simulink model "IntegrationTestSim"  (R2018b)
settings: Solver=ode45  StartTime=0.0  StopTime=600  RelTol=1e-3  EnableMultiTasking=on
values from neighbouring files (symbols this model uses):
  enableHorzMan = 1    [IntegrationTestClass.m]
  enableVertMan = 0    [IntegrationTestClass.m]
  ignorePrevAlert = 1    [IntegrationTestClass.m]
  sim_sampleTime = 0.1    [IntegrationTestClass.m]
  uasSensorSelected = 1    [IntegrationTestClass.m]
  uasSurveillance_sampleTime = 0.1    [IntegrationTestClass.m]
undefined symbols (not defined in the file or in its folder): ac1dyn_alt0_ft, ac1dyn_lat0_rad, ac1dyn_lon0_rad, daa_turnRate_dps, daa_vertRate_fpm, dh_flag, dh_ftps, dpsi_flag, dpsi_radps, uasPilot_altitudeK, uasPilot_altitudeOffset, uasPilot_altitudeTheta, uasPilot_coordDelayK, uasPilot_coordDelayMin, uasPilot_coordDelayTheta, uasPilot_desiredTurnRate_dps, uasPilot_desiredVertRate_ftpm, uasPilot_deterministicMode, uasPilot_dt_s, uasPilot_executionDelayMin, uasPilot_executionDelayMu, uasPilot_initialDelayMin, uasPilot_initialDelayMu, uasPilot_maxRelativeHdg, uasPilot_meanUpdateTimes, uasPilot_mentalFilter_climbThresh_fps, uasPilot_mentalFilter_numSamp, uasPilot_mentalFilter_turnThresh_rad, uasPilot_minUpdateTimes, uasPilot_operatorEnabled, uasPilot_probDescend, uasPilot_probFollowMinDev, uasPilot_probLeftTurn, uasPilot_probTurn, uasPilot_reducedClimbAlt_ft, uasPilot_reducedTurnAngle_deg, uasPilot_seedChoose, uasPilot_seedCoordDelay, uasPilot_seedExecutionDelay, uasPilot_seedInitialDelay, uasPilot_seedTurn, uasPilot_seedUpdate, uasPilot_seedVertical, uasPilot_triggerLevel, uasPilot_turnK, uasPilot_turnOffset, uasPilot_turnTheta
libraries: simulink x4, BasicAircraftDynamicsBlock x3, NominalTrajectory x2, FlattenAircraftEstimateBus x2, PerfectSurveillanceBlock x2, sph2cart x2, DaidalusV201Block x1, HysteresisFilterBlock x1, MofNFilterBlock x1, CommonMetricsBlock x1, SLoWCBlock x1, WellClearMetricsBlock x1
(part 1 of 3)
settings Model: Creator=JO20596  LastModifiedBy=BI28030
settings DataIOCC: LimitDataPoints=on  MaxDataPoints=10000  SignalLoggingSaveFormat=ModelDataLogs  SaveState=on  StateSaveName=xoutNew  OutputSaveName=youtNew
settings OptimizationCC: ExpressionDepthLimit=2147483647  LifeSpan=inf
settings DebuggingCC: UnderspecifiedInitializationDetection=Classic  MergeDetectMultiDrivingBlocksExec=none  SolverPrmCheckMsg=warning  FcnCallInpInsideContextMsg=warning  StateNameClashWarn=warning  SFUnexpectedBacktrackingDiag=warning  SFNoUnconditionalDefaultTransitionDiag=warning  SFExecutionAtInitializationDiag=none
settings HardwareCC: ProdBitPerPointer=32  ProdBitPerSizeT=32  ProdBitPerPtrDiffT=32  ProdLargestAtomicFloat=None  ProdIntDivRoundTo=Undefined  ProdEndianess=Unspecified  ProdWordSize=32  ProdHWDeviceType=32-bit Generic
settings ModelReferenceCC: PropagateSignalLabelsOutOfModel=off
settings SFSimCC: SimUseLocalCustomCode=off
settings RTWCC: RTWUseLocalCustomCode=off
settings CodeAppCC: StateflowObjectComments=on
settings GRTTargetCC: TargetLangStandard=C89/C90 (ANSI)  GeneratePreprocessorConditionals=Disable all  CombineOutputUpdateFcns=off  GRTInterface=on
settings ConfigComp: CovMetricSettings=dw  CovHtmlReporting=on  CovSaveCumulativeToWorkspaceVar=on  CovSaveSingleToWorkspaceVar=on  CovExternalEMLEnable=off

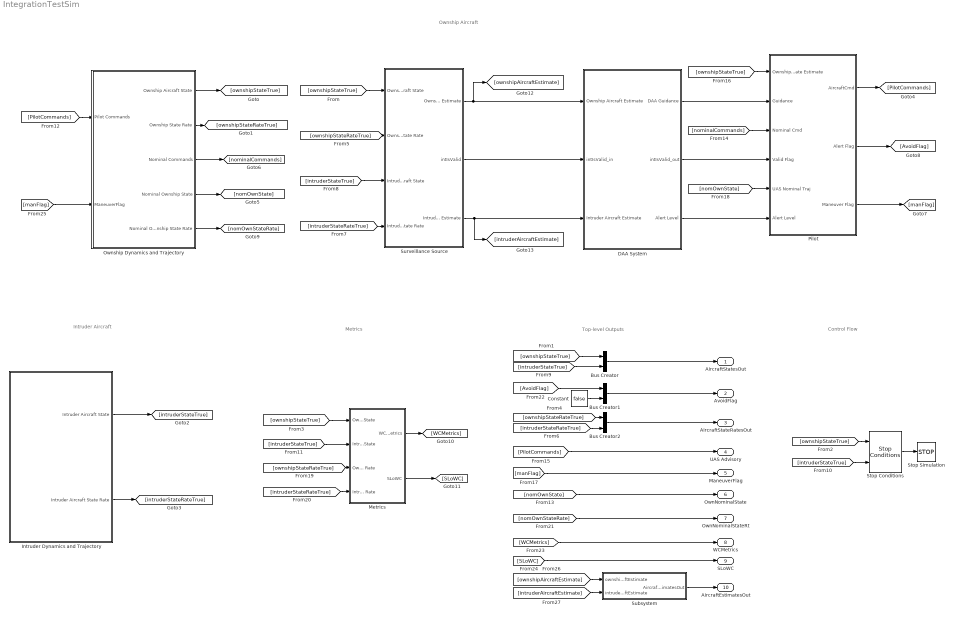
== system IntegrationTestSim ==
  note: Metrics
  note: Control Flow
  note: Top-level Outputs
  note: Ownship Aircraft
  note: Intruder Aircraft
  Bus Creator : BusCreator  Inputs=2
  Bus Creator1 : BusCreator  Inputs=2
  Bus Creator2 : BusCreator  Inputs=2
  Constant : Constant  Value=false  SampleTime=sim_sampleTime
  DAA System : Subsystem
  Intruder Dynamics and Trajectory : Subsystem
  Metrics : Subsystem
  Ownship Dynamics and Trajectory : Subsystem
  Pilot : Subsystem  mask(Heuristic Operator Model){dt=uasPilot_dt_s, operator_enabled=uasPilot_operatorEnabled, deterministicMode=uasPilot_deterministicMode, trigger_level=uasPilot_triggerLevel, mean_initial_delay=uasPilot_initialDelayMu, min_initial_delay=uasPilot_initialDelayMin, coord_delay_k=uasPilot_coordDelayK, coord_delay_theta=uasPilot_coordDelayTheta, coord_delay_min=uasPilot_coordDelayMin, mean_exec_delay=uasPilot_executionDelayMu, min_exec_delay=uasPilot_executionDelayMin, min_upd_times=uasPilot_minUpdateTimes, mean_upd_times=uasPilot_meanUpdateTimes, rng_seed_initial=uasPilot_seedInitialDelay, rng_seed_coord=uasPilot_seedCoordDelay, rng_seed_execution=uasPilot_seedExecutionDelay, rng_seed_update=uasPilot_seedUpdate, prob_follow_min=uasPilot_probFollowMinDev, prob_turn_left=uasPilot_probLeftTurn, prob_descend=uasPilot_probDescend, prob_turn=uasPilot_probTurn, max_hdg_diff=uasPilot_maxRelativeHdg, turn_k=uasPilot_turnK, turn_theta=uasPilot_turnTheta, turn_offset=uasPilot_turnOffset, alt_k=uasPilot_altitudeK, alt_theta=uasPilot_altitudeTheta, alt_offset=uasPilot_altitudeOffset, rng_seed_horz=uasPilot_seedTurn, rng_seed_vert=uasPilot_seedVertical, rng_seed_horz_vs_vert=uasPilot_seedChoose, max_turn_rate=uasPilot_desiredTurnRate_dps, settle_angle=uasPilot_reducedTurnAngle_deg, max_vert_rate=uasPilot_desiredVertRate_ftpm, settle_dist=uasPilot_reducedClimbAlt_ft, mental_filter_samples=uasPilot_mentalFilter_numSamp, mental_filter_turn_thresh=uasPilot_mentalFilter_turnThresh_rad, mental_filter_climb_thresh=uasPilot_mentalFilter_climbThresh_fps, daa_turnRate=daa_turnRate_dps, daa_vertRate=daa_vertRate_fpm}
      mask prompts: dt "Sample Time"; operator_enabled "Enable Pilot Response?"; deterministicMode "Deterministic Mode?"; trigger_level "Trigger Alert Level"; mean_initial_delay "Mean Initial Delay"; min_initial_delay "Minimum Initial Delay"; coord_delay_k "Coordination Delay Shape Parameter (k)"; coord_delay_theta "Coordination Delay Scale Parameter (theta)"; coord_delay_min "Minimum Coordination Delay"; mean_exec_delay "Mean Execution Delay"; min_exec_delay "Minimum Execution Delay"; min_upd_times "Minimum Maneuver Update Times by Alert Level"; mean_upd_times "Mean Maneuver Update Times by Alert Level (sec)"; rng_seed_initial "Random Seed (Initial Delay)"; rng_seed_coord "Random Seed (Coordiantion Delay)"; rng_seed_execution "Random Seed (Execution Delay)"; rng_seed_update "Random Seed (Update Decision)"; prob_follow_min "Probability of Following Minimum Turn"; prob_turn_left "Probability of Turning Left vs. Right"; prob_descend "Probability of Descend vs. CLimb"; prob_turn "Probability of Choosing Turn"; max_hdg_diff "Maximum Heading Difference to Override"; turn_k "Turn Magnitude Shape Parameter (k)"; turn_theta "Turn Magnitude Scale Parameter (theta)"; turn_offset "Turn Magnitude Offset"; alt_k "Altitude Shape Parameter (k)"; alt_theta "Altitude Scale Parameter (theta)"; alt_offset "Altitude Offset"; rng_seed_horz "Random Seed (Horizontal Maneuver Choice)"; rng_seed_vert "Random Seed (Vertical Maneuver Choice)"; rng_seed_horz_vs_vert "Random Seed (Turn vs. Climb)"; max_turn_rate "Desired Turn Rate (deg/s)"; settle_angle "Angle from Desired Heading to Begin Settle (deg)"; max_vert_rate "Desired Vertical Rate (ft/min)"; settle_dist "Distance from Desired Altitude to Begin Settle (ft)"; mental_filter_samples "Number of Samples for Mental Filter"; mental_filter_turn_thresh "Mental Filter Turn Threshold (rad)"; mental_filter_climb_thresh "Mental Filter Climb Threshold (fps)"; daa_turnRate "Max Turn Rate (deg/s)"; daa_vertRate "Max Vertical Rate (fpm)"
      mask help: Identifies pilot response to surveillance estimates of intruder position/course. Either a horizontal or vertical maneuver to maintain well clear.
      mask DialogControl ParameterTabVar0 Prompt: Tab
      mask DialogControl ParameterTabVar01 Prompt: Alert
      mask DialogControl ParameterTabVar012 Prompt: Maneuver Timing
      mask DialogControl ParameterTabVar0123 Prompt: Maneuver Selection
      mask DialogControl ParameterTabVar01234 Prompt: Maneuver Dynamics
      mask DialogControl Container12 Prompt: Pilot Mental Filter
      mask DialogControl Container11 Prompt: DAIDALUS Parameters
  Stop Conditions : StopConditionsBlock/Stop Conditions  range_limit_ft=stop_range_ft  altitude_limit_ft=stop_altitude_ft
  Stop Simulation : Stop
  Subsystem : Subsystem
  Surveillance Source : Subsystem
  AircraftStatesOut : Outport
  AvoidFlag : Outport  Port=2
  AircraftStateRatesOut : Outport  Port=3
  UAS Advisory : Outport  Port=4
  ManeuverFlag : Outport  Port=5
  OwnNominalState : Outport  Port=6
  OwnNominalStateRt : Outport  Port=7
  WCMetrics : Outport  Port=8
  SLoWC : Outport  Port=9
  AircraftEstimatesOut : Outport  Port=10
  wires:
  Bus Creator1/1 -> AvoidFlag/1
  Bus Creator2/1 -> AircraftStateRatesOut/1
  Constant/1 -> Bus Creator1/2
  [AvoidFlag] -> Bus Creator1/1
  Stop Conditions/1 -> Stop Simulation/1
  Bus Creator/1 -> AircraftStatesOut/1
  [ownshipStateTrue] -> Surveillance Source/1(Ownship Aircraft State)
  [ownshipStateTrue] -> Bus Creator/1
  [ownshipStateTrue] -> Stop Conditions/1
  [ownshipStateRateTrue] -> Bus Creator2/1
  [ownshipStateRateTrue] -> Surveillance Source/2(Ownship Aircraft State Rate)
  [intruderStateRateTrue] -> Bus Creator2/2
  [intruderStateRateTrue] -> Surveillance Source/4(Intruder Aircraft State Rate)
  [intruderStateTrue] -> Surveillance Source/3(Intruder Aircraft State)
  [intruderStateTrue] -> Bus Creator/2
  [intruderStateTrue] -> Stop Conditions/2
  Pilot/1(AircraftCmd) -> [PilotCommands]
  DAA System/1(DAA Guidance) -> Pilot/2(Guidance)
  DAA System/3(Alert Level) -> Pilot/6(Alert Level)
  [nomOwnState] -> Pilot/5(UAS Nominal Traj)
  [nominalCommands] -> Pilot/3(Nominal Cmd)
  DAA System/2(intIsValid_out) -> Pilot/4(Valid Flag)
  Surveillance Source/1(Ownship Aircraft Estimate) -> [ownshipAircraftEstimate], DAA System/1(Ownship Aircraft Estimate)
  Surveillance Source/2(intIsValid) -> DAA System/2(intIsValid_in)
  Surveillance Source/3(Intruder Aircraft Estimate) -> [intruderAircraftEstimate], DAA System/3(Intruder Aircraft Estimate)
  [ownshipStateTrue] -> Pilot/1(Ownship State Estimate)
  [PilotCommands] -> UAS Advisory/1
  Pilot/3(Maneuver Flag) -> [manFlag]
  [manFlag] -> ManeuverFlag/1
  [ownshipStateTrue] -> Metrics/1(Ownship State)
  [intruderStateTrue] -> Metrics/2(Intruder State)
  Pilot/2(Alert Flag) -> [AvoidFlag]
  [ownshipStateRateTrue] -> Metrics/3(Ownship State Rate)
  [intruderStateRateTrue] -> Metrics/4(Intruder State Rate)
  [nomOwnState] -> OwnNominalState/1
  [nomOwnStateRate] -> OwnNominalStateRt/1
  Metrics/1(WCMetrics) -> [WCMetrics]
  Metrics/2(SLoWC) -> [SLoWC]
  [WCMetrics] -> WCMetrics/1
  [SLoWC] -> SLoWC/1
  [PilotCommands] -> Ownship Dynamics and Trajectory/1(Pilot Commands)
  Ownship Dynamics and Trajectory/1(Ownship Aircraft State) -> [ownshipStateTrue]
  Ownship Dynamics and Trajectory/2(Ownship State Rate) -> [ownshipStateRateTrue]
  Ownship Dynamics and Trajectory/3(Nominal Commands) -> [nominalCommands]
  Ownship Dynamics and Trajectory/4(Nominal Ownship State) -> [nomOwnState]
  Ownship Dynamics and Trajectory/5(Nominal Ownship State Rate) -> [nomOwnStateRate]
  Intruder Dynamics and Trajectory/1(Intruder Aircraft State) -> [intruderStateTrue]
  Intruder Dynamics and Trajectory/2(Intruder Aircraft State Rate) -> [intruderStateRateTrue]
  [manFlag] -> Ownship Dynamics and Trajectory/2(ManeuverFlag)
  [ownshipAircraftEstimate] -> Subsystem/1(ownshipAircraftEstimate)
  [intruderAircraftEstimate] -> Subsystem/2(intruderAircraftEstimate)
  Subsystem/1(AircraftEstimatesOut) -> AircraftEstimatesOut/1

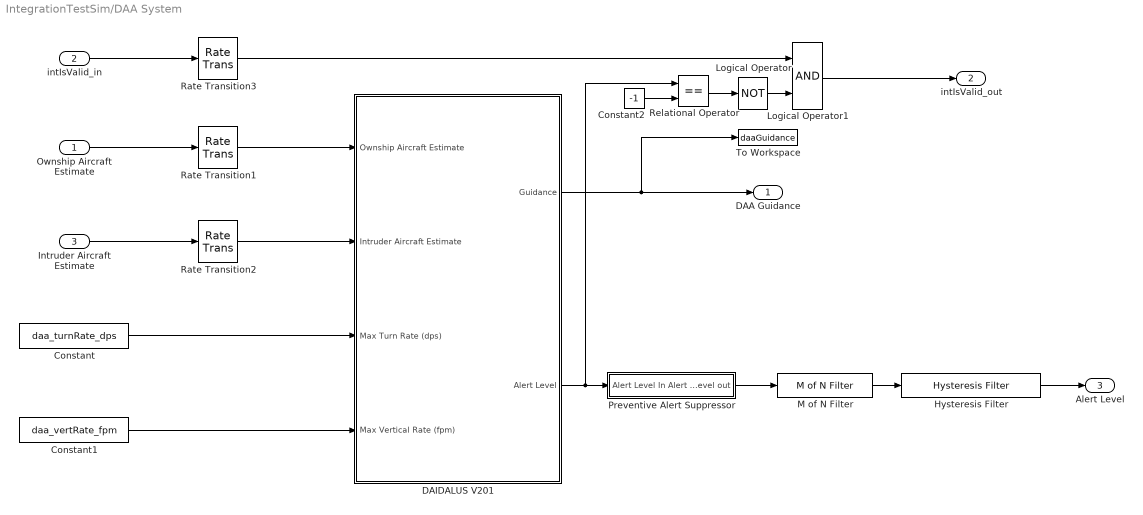
== system IntegrationTestSim/DAA System ==
  Ownship Aircraft Estimate : Inport
  intIsValid_in : Inport  Port=2
  Intruder Aircraft Estimate : Inport  Port=3
  Constant : Constant  Value=daa_turnRate_dps
  Constant1 : Constant  Value=daa_vertRate_fpm
  Constant2 : Constant  Value=-1
  DAIDALUS V201 : Subsystem
  Hysteresis Filter : HysteresisFilterBlock/Hysteresis Filter  signal_hold_time=ac1AlertHyst_signalHoldTime
  Logical Operator : Logic  Operator=NOT  AllPortsSameDT=off  OutDataTypeStr=boolean
  Logical Operator1 : Logic  AllPortsSameDT=off  OutDataTypeStr=boolean
  M of N Filter : MofNFilterBlock/M of N Filter  num_samples=ac1AlertMofN_numSamples  num_upgrade=ac1AlertMofN_numSamplesUp  num_downgrade=ac1AlertMofN_numSamplesDown
  Preventive Alert Suppressor : Subsystem
  Rate Transition1 : RateTransition  OutPortSampleTime=uasLogic_sampleTime
  Rate Transition2 : RateTransition  OutPortSampleTime=uasLogic_sampleTime
  Rate Transition3 : RateTransition  OutPortSampleTime=uasLogic_sampleTime
  Relational Operator : RelationalOperator  Operator===  OutDataTypeStr=boolean  RndMeth=Simplest
  To Workspace : ToWorkspace  VariableName=daaGuidance  SampleTime=-1
  DAA Guidance : Outport
  intIsValid_out : Outport  Port=2
  Alert Level : Outport  Port=3
  wires:
  Ownship Aircraft Estimate/1 -> Rate Transition1/1
  Intruder Aircraft Estimate/1 -> Rate Transition2/1
  DAIDALUS V201/2(Alert Level) -> Relational Operator/1, Preventive Alert Suppressor/1(Alert Level In)
  Constant/1 -> DAIDALUS V201/3(Max Turn Rate (dps))
  Constant1/1 -> DAIDALUS V201/4(Max Vertical Rate (fpm))
  DAIDALUS V201/1(Guidance) -> To Workspace/1, DAA Guidance/1
  Hysteresis Filter/1 -> Alert Level/1
  Preventive Alert Suppressor/1(Alert Level out) -> M of N Filter/1
  intIsValid_in/1 -> Rate Transition3/1
  Rate Transition1/1 -> DAIDALUS V201/1(Ownship Aircraft Estimate)
  Rate Transition2/1 -> DAIDALUS V201/2(Intruder Aircraft Estimate)
  M of N Filter/1 -> Hysteresis Filter/1
  Constant2/1 -> Relational Operator/2
  Relational Operator/1 -> Logical Operator/1
  Logical Operator/1 -> Logical Operator1/2
  Logical Operator1/1 -> intIsValid_out/1
  Rate Transition3/1 -> Logical Operator1/1

== system IntegrationTestSim/Intruder Dynamics and Trajectory ==
  AC2 - Nominal Trajectory : NominalTrajectory/Nominal Trajectory  eventFilename=event2.mat  ts=.1
  Basic Aircraft Dynamics : BasicAircraftDynamicsBlock/Basic Aircraft Dynamics  ts_dynamics=.1  v_ftps_0=ac2dyn_v_ftps  N_ft_0=ac2dyn_N_ft  E_ft_0=ac2dyn_E_ft  h_ft_0=ac2dyn_h_ft  psi_rad_0=ac2dyn_psi_rad  theta_rad_0=ac2dyn_theta_rad  phi_rad_0=ac2dyn_phi_rad  a_ftpss_0=ac2dyn_a_ftpss  v_ftps_max=ac2dyn_con.maxAirspeed_ftps  v_ftps_min=ac2dyn_con.minAirspeed_ftps  dv_ftpss_max=ac2dyn_con.maxAcceleration_ftpss  dv_ftpss_min=ac2dyn_con.minAcceleration_ftpss  dh_ftps_max=ac2dyn_con.maxVerticalRate_ftps  dh_ftps_min=ac2dyn_con.minVerticalRate_ftps  q_radps_max=ac2dyn_con.maxPitchRate_radps  phi_rad_max=ac2dyn_con.maxBankAngle_rad  dphi_radps_max=ac2dyn_con.maxRollRate_radps  r_radps_max=ac2dyn_con.maxYawRate_radps  pNUM=ac2dyn_con.dynamicsNumeratorRollRate  pDEN=ac2dyn_con.dynamicsDenominatorRollRate  hNUM=ac2dyn_con.dynamicsNumeratorVerticalRate  hDEN=ac2dyn_con.dynamicsDenominatorVerticalRate  rNUM=ac2dyn_con.dynamicsNumeratorYawRate  rDEN=ac2dyn_con.dynamicsDenominatorYawRate  lat0_rad=ac2dyn_lat0_rad  lon0_rad=ac2dyn_lon0_rad  alt_ft=ac2dyn_alt0_ft
  Terminator1 : Terminator
  Intruder Aircraft State : Outport
  Intruder Aircraft State Rate : Outport  Port=2
  wires:
  Basic Aircraft Dynamics/2 -> Terminator1/1
  Basic Aircraft Dynamics/1 -> Intruder Aircraft State/1  "Aircraft2"
  AC2 - Nominal Trajectory/1 -> Basic Aircraft Dynamics/1
  Basic Aircraft Dynamics/3 -> Intruder Aircraft State Rate/1

== system IntegrationTestSim/Metrics ==
  Ownship State : Inport
  Intruder State : Inport  Port=2
  Ownship State Rate : Inport  Port=3
  Intruder State Rate : Inport  Port=4
  Common Metrics : CommonMetricsBlock/Common Metrics
  Compute SLoWC : Subsystem  mask{DMOD=4000, tauMod=35, altDiff=450}
      mask prompts: altDiff "Altitude Difference Threshold:"
  Well Clear Metrics : Subsystem
  WCMetrics : Outport
  SLoWC : Outport  Port=2
  wires:
  Ownship State/1 -> Common Metrics/1, Well Clear Metrics/1(ownState), Compute SLoWC/1(ownState)
  Intruder State/1 -> Common Metrics/2, Well Clear Metrics/2(intState), Compute SLoWC/2(intState)
  Ownship State Rate/1 -> Well Clear Metrics/3(ownStateRate), Compute SLoWC/3(ownStateRate)
  Intruder State Rate/1 -> Well Clear Metrics/4(intStateRate), Compute SLoWC/4(intStateRate)
  Well Clear Metrics/1(WCV_MIT) -> WCMetrics/1
  Compute SLoWC/1(SLoWC) -> SLoWC/1

== system IntegrationTestSim/Ownship Dynamics and Trajectory ==
  Pilot Commands : Inport
  ManeuverFlag : Inport  Port=2
  Basic Aircraft Dynamics : BasicAircraftDynamicsBlock/Basic Aircraft Dynamics  ts_dynamics=.1  v_ftps_0=ac1dyn_v_ftps  N_ft_0=ac1dyn_N_ft  E_ft_0=ac1dyn_E_ft  h_ft_0=ac1dyn_h_ft  psi_rad_0=ac1dyn_psi_rad  theta_rad_0=ac1dyn_theta_rad  phi_rad_0=ac1dyn_phi_rad  a_ftpss_0=ac1dyn_a_ftpss  v_ftps_max=ac1dyn_con.maxAirspeed_ftps  v_ftps_min=ac1dyn_con.minAirspeed_ftps  dv_ftpss_max=ac1dyn_con.maxAcceleration_ftpss  dv_ftpss_min=ac1dyn_con.minAcceleration_ftpss  dh_ftps_max=ac1dyn_con.maxVerticalRate_ftps  dh_ftps_min=ac1dyn_con.minVerticalRate_ftps  q_radps_max=ac1dyn_con.maxPitchRate_radps  phi_rad_max=ac1dyn_con.maxBankAngle_rad  dphi_radps_max=ac1dyn_con.maxRollRate_radps  r_radps_max=ac1dyn_con.maxYawRate_radps  pNUM=ac1dyn_con.dynamicsNumeratorRollRate  pDEN=ac1dyn_con.dynamicsDenominatorRollRate  hNUM=ac1dyn_con.dynamicsNumeratorVerticalRate  hDEN=ac1dyn_con.dynamicsDenominatorVerticalRate  rNUM=ac1dyn_con.dynamicsNumeratorYawRate  rDEN=ac1dyn_con.dynamicsDenominatorYawRate  lat0_rad=ac2dyn_lat0_rad  lon0_rad=ac2dyn_lon0_rad  alt_ft=ac2dyn_alt0_ft
  Multiport Switch : MultiPortSwitch  DataPortOrder=Specify indices  DataPortIndices={1,0}
  Nominal Commands and Trajectory : Subsystem
  Terminator : Terminator
  Ownship Aircraft State : Outport
  Ownship State Rate : Outport  Port=2
  Nominal Commands : Outport  Port=3
  Nominal Ownship State : Outport  Port=4
  Nominal Ownship State Rate : Outport  Port=5
  wires:
  Nominal Commands and Trajectory/3(NominalOwnshipStateRate) -> Nominal Ownship State Rate/1
  Basic Aircraft Dynamics/1 -> Ownship Aircraft State/1  "Aircraft1"
  Nominal Commands and Trajectory/1(Nominal Commands) -> Nominal Commands/1, Multiport Switch/3
  Basic Aircraft Dynamics/3 -> Ownship State Rate/1
  Nominal Commands and Trajectory/2(NominalOwnshipState) -> Nominal Ownship State/1
  Basic Aircraft Dynamics/2 -> Terminator/1
  ManeuverFlag/1 -> Multiport Switch/1
  Multiport Switch/1 -> Basic Aircraft Dynamics/1
  Pilot Commands/1 -> Multiport Switch/2

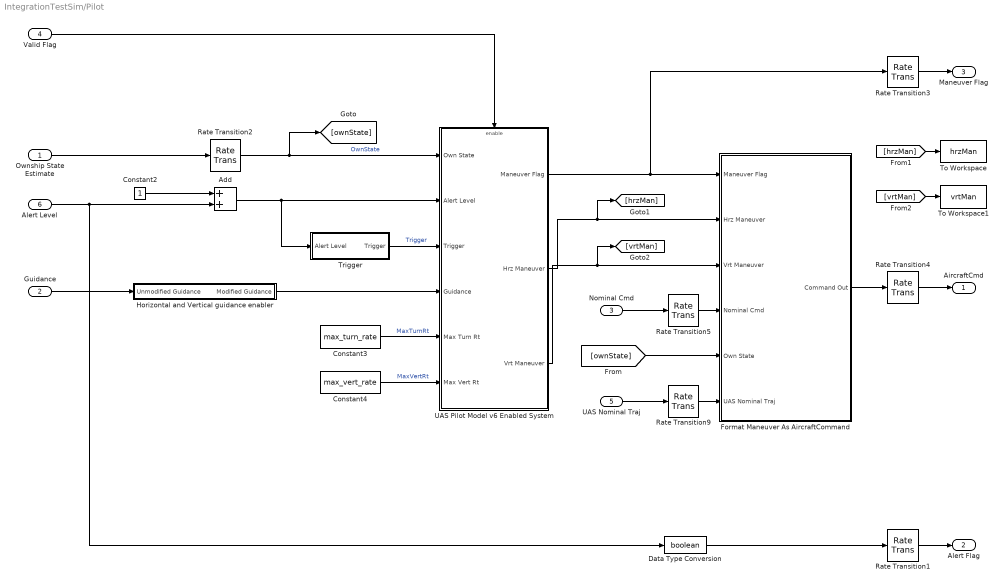
== system IntegrationTestSim/Pilot ==
  Ownship State Estimate : Inport
  Guidance : Inport  Port=2
  Nominal Cmd : Inport  Port=3
  Valid Flag : Inport  Port=4
  UAS Nominal Traj : Inport  Port=5
  Alert Level : Inport  Port=6
  Add : Sum
  Constant2 : Constant
  Constant3 : Constant  Value=max_turn_rate
  Constant4 : Constant  Value=max_vert_rate
  Data Type Conversion : DataTypeConversion  OutDataTypeStr=boolean
  Format Maneuver As AircraftCommand : Subsystem
  Horizontal and Vertical guidance enabler : Subsystem
  Rate Transition1 : RateTransition  OutPortSampleTime=0.1
  Rate Transition2 : RateTransition  OutPortSampleTime=1
  Rate Transition3 : RateTransition  OutPortSampleTime=0.1
  Rate Transition4 : RateTransition  OutPortSampleTime=0.1
  Rate Transition5 : RateTransition  OutPortSampleTime=1
  Rate Transition9 : RateTransition  OutPortSampleTime=1
  To Workspace : ToWorkspace  VariableName=hrzMan  SaveFormat=Timeseries  SampleTime=-1
  To Workspace1 : ToWorkspace  VariableName=vrtMan  SaveFormat=Timeseries  SampleTime=-1
  Trigger : Subsystem  mask{trigger_level=trigger_level}
      mask prompts: trigger_level "Alert Level for Trigger"
      mask DialogControl Container6 Prompt: M of N Filter Parameters
      mask DialogControl Container7 Prompt: Hysteresis Parameters
  UAS Pilot Model v6 Enabled System : Subsystem
  AircraftCmd : Outport
  Alert Flag : Outport  Port=2
  Maneuver Flag : Outport  Port=3
  wires:
  Rate Transition1/1 -> Alert Flag/1
  Ownship State Estimate/1 -> Rate Transition2/1
  Rate Transition3/1 -> Maneuver Flag/1
  Nominal Cmd/1 -> Rate Transition5/1
  UAS Pilot Model v6 Enabled System/1(Maneuver Flag) -> Format Maneuver As AircraftCommand/1(Maneuver Flag), Rate Transition3/1
  [ownState] -> Format Maneuver As AircraftCommand/5(Own State)
  Format Maneuver As AircraftCommand/1(Command Out) -> Rate Transition4/1
  Rate Transition5/1 -> Format Maneuver As AircraftCommand/4(Nominal Cmd)
  Rate Transition2/1 -> UAS Pilot Model v6 Enabled System/1(Own State), [ownState]  "OwnState"
  UAS Pilot Model v6 Enabled System/2(Hrz Maneuver) -> [hrzMan], Format Maneuver As AircraftCommand/2(Hrz Maneuver)
  Constant2/1 -> Add/1
  Constant3/1 -> UAS Pilot Model v6 Enabled System/5(Max Turn Rt)  "MaxTurnRt"
  Constant4/1 -> UAS Pilot Model v6 Enabled System/6(Max Vert Rt)  "MaxVertRt"
  Data Type Conversion/1 -> Rate Transition1/1
  Trigger/1(Trigger) -> UAS Pilot Model v6 Enabled System/3(Trigger)  "Trigger"
  Valid Flag/1 -> UAS Pilot Model v6 Enabled System/Enable
  Guidance/1 -> Horizontal and Vertical guidance enabler/1(Unmodified Guidance)
  UAS Pilot Model v6 Enabled System/3(Vrt Maneuver) -> [vrtMan], Format Maneuver As AircraftCommand/3(Vrt Maneuver)
  Horizontal and Vertical guidance enabler/1(Modified Guidance) -> UAS Pilot Model v6 Enabled System/4(Guidance)
  Alert Level/1 -> Data Type Conversion/1, Add/2
  Rate Transition4/1 -> AircraftCmd/1
  Add/1 -> UAS Pilot Model v6 Enabled System/2(Alert Level), Trigger/1(Alert Level)
  UAS Nominal Traj/1 -> Rate Transition9/1
  Rate Transition9/1 -> Format Maneuver As AircraftCommand/6(UAS Nominal Traj)
  [hrzMan] -> To Workspace/1
  [vrtMan] -> To Workspace1/1

== system IntegrationTestSim/Subsystem ==
  ownshipAircraftEstimate : Inport
  intruderAircraftEstimate : Inport  Port=2
  Bus Creator : BusCreator  Inputs=2
  Flatten AircraftEstimate Bus : FlattenAircraftEstimateBus/Flatten AircraftEstimate Bus  SystemSampleTime=-1
  Flatten AircraftEstimate Bus1 : FlattenAircraftEstimateBus/Flatten AircraftEstimate Bus  SystemSampleTime=-1
  AircraftEstimatesOut : Outport
  wires:
  ownshipAircraftEstimate/1 -> Flatten AircraftEstimate Bus/1
  intruderAircraftEstimate/1 -> Flatten AircraftEstimate Bus1/1
  Flatten AircraftEstimate Bus/1 -> Bus Creator/1
  Flatten AircraftEstimate Bus1/1 -> Bus Creator/2
  Bus Creator/1 -> AircraftEstimatesOut/1

== system IntegrationTestSim/Surveillance Source ==
  Ownship Aircraft State : Inport
  Ownship Aircraft State Rate : Inport  Port=2
  Intruder Aircraft State : Inport  Port=3
  Intruder Aircraft State Rate : Inport  Port=4
  Bus Selector : BusSelector  OutputSignals=isValid
  Ownship Sensor - Perfect Surveillance : PerfectSurveillanceBlock/Perfect Surveillance  Description=|  dt=ac1OwnPerfSurv_surveillanceSampletime_s
      | Documentation for Perfect Observation Block                                                                                                                                                                                                                                                                                                                                                                                                          
      |                                                                                                                                                                                                                                                                                                                                                                                                                                                      
      | Description:  The perfect observation block, also known as a perfect                                                                                                                                                                                                                                                                                                                                                                                 
      | surveillance block, receives an Aircraft State, nominally from a Basic                                                                                                                                                                                                                                                                                                                                                                               
      | Aircraft Dynamics block, and outputs an Aircraft Estimate.  The Aircraft                                                                                                                                                                                                                                                                                                                                                                             
      | State that is received as input consists of Latitude, Longitude, and                                                                                                                                                                                                                                                                                                                                                                                 
      | Altitude state information as well as the aircraft position in local                                                                                                                                                                                                                                                                                                                                                                                 
      | coordinates in units of feet for north, east, and height.  The Aircraft                                                                                                                                                                                                                                                                                                                                                                              
      | Estimate outputs consist of estimates for the aircraft Latitude, Longitude, and Altitude, the east, north up position, and sensor covariance.  For perfect surveillance, the covariance estimates are all set to zero as default.  In addition, "time of validity" and a Boolean flag for the sensor report, "is Valid", are outputted as part of the Aircraft Estimate.                                                                             
      |                                                                                                                                                                                                                                                                                                                                                                                                                                                      
      | The initial perfect surveillance block developed receives the aircraft state information from the "AC2 - Basic Aircraft Dynamics" block within the "nominalEncounter" study.  Since the expected output from the AC1 and AC2 aircraft states have slightly different output parameters than what is provided from the perfect surveillance block (i.e., covariance estimates, isValid, and time of validity), the perfect surveillance block         
      | AircraftEstimate output has been left disconnected.                                                                                                                                                                                                                                                                                                                                                                                                  
      |                                                                                                                                                                                                                                                                                                                                                                                                                                                      
      | The initial unit test performed for this perfect observation block was to                                                                                                                                                                                                                                                                                                                                                                            
      | run the nominalEncounter study and to ensure that the simulation completes and no exceptions are encountered.  This unit test was successful (other than receiving a warning that the output of the perfect surveillance block is not connected, which was expected).  A more comprehensive future unit test would be to evaluate the position inputs and compare them with the position outputs to ensure that they are consistent with one another.
  Subsystem : Subsystem
  Terminator : Terminator
  Ownship Aircraft Estimate : Outport
  intIsValid : Outport  Port=2
  Intruder Aircraft Estimate : Outport  Port=3
  wires:
  Ownship Sensor - Perfect Surveillance/1 -> Ownship Aircraft Estimate/1
  Bus Selector/1 -> intIsValid/1  "<isValid>"
  Subsystem/1(Intruder Aircraft Estimate) -> Bus Selector/1, Intruder Aircraft Estimate/1
  Ownship Sensor - Perfect Surveillance/2 -> Terminator/1
  Ownship Aircraft State/1 -> [ownState]
  Intruder Aircraft State/1 -> Subsystem/3(Intruder Aircraft State)
  Intruder Aircraft State Rate/1 -> Subsystem/4(Intruder Aircraft State Rate)
  [ownState] -> Ownship Sensor - Perfect Surveillance/1
  Ownship Aircraft State Rate/1 -> [ownStateRate]
  [ownStateRate] -> Ownship Sensor - Perfect Surveillance/2
  [ownStateRate] -> Subsystem/2(Ownship Aircraft State Rate)
  [ownState] -> Subsystem/1(Ownship Aircraft State)

== system IntegrationTestSim/DAA System/DAIDALUS V201 ==
  Ownship Aircraft Estimate : Inport
  Intruder Aircraft Estimate : Inport  Port=2
  Max Turn Rate (dps) : Inport  Port=3
  Max Vertical Rate (fpm) : Inport  Port=4
  DAIDALUSv201 : DaidalusV201Block/DAIDALUSv201  DTHR=daa_guideDTHR  ZTHR=daa_guideZTHR  TTHR=daa_guideTTHR  TCOA=daa_guideTCOA  lookahead_time=daa_guideLookahead  use_single_direction=daa_singleDirRecovery  prev_DTHR=daa_prevDTHR  prev_ZTHR=daa_prevZTHR  prev_TTHR=daa_prevTTHR  prev_TCOA=daa_prevTCOA  prev_lookahead=daa_prevLookahead  prev_early=daa_prevEarly  corr_DTHR=daa_corrDTHR  corr_ZTHR=daa_corrZTHR  corr_TTHR=daa_corrTTHR  corr_TCOA=daa_corrTCOA  corr_lookahead=daa_corrLookahead  corr_early=daa_corrEarly  warn_DTHR=daa_warnDTHR  warn_ZTHR=daa_warnZTHR  warn_TTHR=daa_warnTTHR  warn_TCOA=daa_warnTCOA  warn_lookahead=daa_warnLookahead  warn_early=daa_warnEarly  min_alt=daa_minAlt  rec_stab_time=daa_recStabTime  min_hor_rec=daa_minHorRec  ca_factor=daa_caFactor
  Selector : Selector  InputPortWidth=311  IndexOptions=Index vector (dialog)  Indices=[1:283]  OutputSizes=1
  Guidance : Outport
  Alert Level : Outport  Port=2
  wires:
  Ownship Aircraft Estimate/1 -> DAIDALUSv201/1
  DAIDALUSv201/1 -> Selector/1
  Intruder Aircraft Estimate/1 -> DAIDALUSv201/2
  Max Vertical Rate (fpm)/1 -> DAIDALUSv201/4
  DAIDALUSv201/2 -> Alert Level/1
  Max Turn Rate (dps)/1 -> DAIDALUSv201/3
  Selector/1 -> Guidance/1

== system IntegrationTestSim/DAA System/Preventive Alert Suppressor ==
  Alert Level In : Inport
  " " : Constant  Value=0
  "  " : Constant  Value=ignorePrevAlert
  Multiport Switch : MultiPortSwitch  DataPortOrder=Specify indices  DataPortIndices={1,0}
  Multiport Switch1 : MultiPortSwitch  DataPortOrder=Specify indices  DataPortIndices={-1,3,2,1,0}
  Alert Level out : Outport
  wires:
  "  "/1 -> Multiport Switch/1
  Alert Level In/1 -> Multiport Switch/3, Multiport Switch1/3, Multiport Switch1/4, Multiport Switch1/6, Multiport Switch1/1
  " "/1 -> Multiport Switch1/2, Multiport Switch1/5
  Multiport Switch1/1 -> Multiport Switch/2
  Multiport Switch/1 -> Alert Level out/1

== system IntegrationTestSim/Metrics/Compute SLoWC ==
  ownState : Inport
  intState : Inport  Port=2
  ownStateRate : Inport  Port=3
  intStateRate : Inport  Port=4
  SC-228 Severity of Loss of Well Clear Metric : SLoWCBlock/SC-228 Severity of Loss of Well Clear Metric  DMOD=DMOD  altDiffThreshold=altDiff
  SLoWC pre-processing : Subsystem
  SLoWC : Outport
  wires:
  SLoWC pre-processing/2(DH) -> SC-228 Severity of Loss of Well Clear Metric/2
  SC-228 Severity of Loss of Well Clear Metric/1 -> SLoWC/1
  SLoWC pre-processing/1(HMD) -> SC-228 Severity of Loss of Well Clear Metric/1
  ownState/1 -> SLoWC pre-processing/1(Ownship State)
  SLoWC pre-processing/4(Horizontal Proximity) -> SC-228 Severity of Loss of Well Clear Metric/4
  SLoWC pre-processing/3(Range) -> SC-228 Severity of Loss of Well Clear Metric/3
  intState/1 -> SLoWC pre-processing/2(Intruder State)
  intStateRate/1 -> SLoWC pre-processing/4(Intruder State Rate)
  ownStateRate/1 -> SLoWC pre-processing/3(Ownship State Rate)

== system IntegrationTestSim/Metrics/Well Clear Metrics ==
  ownState : Inport  OutDataTypeStr=Bus: AircraftState
  intState : Inport  Port=2  OutDataTypeStr=Bus: AircraftState
  ownStateRate : Inport  Port=3  OutDataTypeStr=Bus: AircraftStateRate
  intStateRate : Inport  Port=4  OutDataTypeStr=Bus: AircraftStateRate
  Bus Selector : BusSelector  OutputSignals=Ndot_ftps,Edot_ftps,hdot_ftps
  Bus Selector1 : BusSelector  OutputSignals=Ndot_ftps,Edot_ftps,hdot_ftps
  Bus Selector2 : BusSelector  OutputSignals=n_ft,e_ft,h_ft
  Bus Selector3 : BusSelector  OutputSignals=n_ft,e_ft,h_ft
  Data Type Conversion : DataTypeConversion  OutDataTypeStr=double
  Mux : Mux  Inputs=6
  Mux1 : Mux  Inputs=6
  Well Clear Metrics : WellClearMetricsBlock/Well Clear Metrics  tauThreshold=wcm_modTau  hmdThreshold=wcm_HMD  tauVThreshold=wcm_TOCA  altThreshold=wcm_altThresh  rngThreshold=wcm_rangeThresh
  WCV_MIT : Outport
  wires:
  Well Clear Metrics/1 -> Data Type Conversion/1
  intStateRate/1 -> Bus Selector/1
  ownStateRate/1 -> Bus Selector1/1
  ownState/1 -> Bus Selector2/1
  intState/1 -> Bus Selector3/1
  Bus Selector3/1 -> Mux/1  "<n_ft>"
  Bus Selector3/2 -> Mux/2  "<e_ft>"
  Bus Selector3/3 -> Mux/3  "<h_ft>"
  Bus Selector/1 -> Mux/4  "<Ndot_ftps>"
  Bus Selector/2 -> Mux/5  "<Edot_ftps>"
  Bus Selector/3 -> Mux/6  "<hdot_ftps>"
  Bus Selector2/1 -> Mux1/1  "<n_ft>"
  Bus Selector2/2 -> Mux1/2  "<e_ft>"
  Bus Selector2/3 -> Mux1/3  "<h_ft>"
  Bus Selector1/3 -> Mux1/6  "<hdot_ftps>"
  Bus Selector1/1 -> Mux1/4  "<Ndot_ftps>"
  Bus Selector1/2 -> Mux1/5  "<Edot_ftps>"
  Mux1/1 -> Well Clear Metrics/1
  Mux/1 -> Well Clear Metrics/2
  Data Type Conversion/1 -> WCV_MIT/1

== system IntegrationTestSim/Ownship Dynamics and Trajectory/Nominal Commands and Trajectory ==
  AC1 - Nominal Trajectory : NominalTrajectory/Nominal Trajectory  eventFilename=event1.mat  ts=.1
  Basic Aircraft Dynamics : BasicAircraftDynamicsBlock/Basic Aircraft Dynamics  ts_dynamics=.1  v_ftps_0=ac1dyn_v_ftps  N_ft_0=ac1dyn_N_ft  E_ft_0=ac1dyn_E_ft  h_ft_0=ac1dyn_h_ft  psi_rad_0=ac1dyn_psi_rad  theta_rad_0=ac1dyn_theta_rad  phi_rad_0=ac1dyn_phi_rad  a_ftpss_0=ac1dyn_a_ftpss  v_ftps_max=ac1dyn_con.maxAirspeed_ftps  v_ftps_min=ac1dyn_con.minAirspeed_ftps  dv_ftpss_max=ac1dyn_con.maxAcceleration_ftpss  dv_ftpss_min=ac1dyn_con.minAcceleration_ftpss  dh_ftps_max=ac1dyn_con.maxVerticalRate_ftps  dh_ftps_min=ac1dyn_con.minVerticalRate_ftps  q_radps_max=ac1dyn_con.maxPitchRate_radps  phi_rad_max=ac1dyn_con.maxBankAngle_rad  dphi_radps_max=ac1dyn_con.maxRollRate_radps  r_radps_max=ac1dyn_con.maxYawRate_radps  pNUM=ac1dyn_con.dynamicsNumeratorRollRate  pDEN=ac1dyn_con.dynamicsDenominatorRollRate  hNUM=ac1dyn_con.dynamicsNumeratorVerticalRate  hDEN=ac1dyn_con.dynamicsDenominatorVerticalRate  rNUM=ac1dyn_con.dynamicsNumeratorYawRate  rDEN=ac1dyn_con.dynamicsDenominatorYawRate  lat0_rad=ac2dyn_lat0_rad  lon0_rad=ac2dyn_lon0_rad  alt_ft=ac2dyn_alt0_ft
  Terminator : Terminator
  Nominal Commands : Outport
  NominalOwnshipState : Outport  Port=2
  NominalOwnshipStateRate : Outport  Port=3
  wires:
  AC1 - Nominal Trajectory/1 -> Basic Aircraft Dynamics/1, Nominal Commands/1
  Basic Aircraft Dynamics/1 -> NominalOwnshipState/1  "Aircraft1"
  Basic Aircraft Dynamics/2 -> Terminator/1
  Basic Aircraft Dynamics/3 -> NominalOwnshipStateRate/1

== system IntegrationTestSim/Pilot/Format Maneuver As AircraftCommand ==
  Maneuver Flag : Inport  OutDataTypeStr=boolean
  Hrz Maneuver : Inport  Port=2
  Vrt Maneuver : Inport  Port=3
  Nominal Cmd : Inport  Port=4  OutDataTypeStr=Bus: AircraftCommands
  Own State : Inport  Port=5  OutDataTypeStr=Bus: AircraftState
  UAS Nominal Traj : Inport  Port=6
  Get Previous Command : Subsystem
  Horizontal Maneuver : Subsystem  TreatAsAtomicUnit=on
  Unit Delay : UnitDelay  SampleTime=-1
  Vertical Maneuver : Subsystem  TreatAsAtomicUnit=on
  Command Out : Outport  OutDataTypeStr=Bus: AircraftCommands
  wires:
  Maneuver Flag/1 -> Vertical Maneuver/4(Maneuver Flag), Horizontal Maneuver/4(Maneuver Flag), Get Previous Command/3(Maneuver Flag)
  Nominal Cmd/1 -> Get Previous Command/2(Nominal Cmd)
  Unit Delay/1 -> Get Previous Command/1(Cmd In)
  Own State/1 -> Vertical Maneuver/3(Own State), Horizontal Maneuver/3(Own State)
  Hrz Maneuver/1 -> Horizontal Maneuver/2(Maneuver)
  Vrt Maneuver/1 -> Vertical Maneuver/2(Maneuver)
  Horizontal Maneuver/1(Cmd Out) -> Vertical Maneuver/1(Command In)
  Vertical Maneuver/1(Cmd Out) -> Command Out/1, Unit Delay/1
  Get Previous Command/1(Cmd Out) -> Horizontal Maneuver/1(Command In)
  UAS Nominal Traj/1 -> Vertical Maneuver/5(UAS Nominal Traj)

== system IntegrationTestSim/Pilot/Horizontal and Vertical guidance enabler ==
  Unmodified Guidance : Inport
  " " : Constant  Value=enableVertMan
  " 1" : Constant  Value=enableHorzMan
  Horizontal Band manipulation : MATLAB Function  TreatAsAtomicUnit=on
  Switch : Switch  Criteria=u2 > Threshold
  Switch1 : Switch  Criteria=u2 > Threshold
  Vertical Band manipulation : MATLAB Function  TreatAsAtomicUnit=on
  Modified Guidance : Outport
  wires:
  " "/1 -> Switch/2
  Vertical Band manipulation/1(Guidance_out) -> Switch/3  "Guidance"
  Unmodified Guidance/1 -> Vertical Band manipulation/1(Guidance_in), Switch/1
  " 1"/1 -> Switch1/2
  Switch/1 -> Switch1/1, Horizontal Band manipulation/1(Guidance_in)
  Switch1/1 -> Modified Guidance/1
  Horizontal Band manipulation/1(Guidance_out) -> Switch1/3

== system IntegrationTestSim/Pilot/Trigger ==
  Alert Level : Inport
  Filter Alerts : Subsystem  AncestorBlock=CABSAA_ModelLibrary/Filter Alerts  mask(Filter Alerts){trigger_level=trigger_level}
      mask prompts: trigger_level "Alert Level for Trigger"
      mask help: Holds alert level for at least the specified time unless the alert level increases.
  Trigger : Outport
  wires:
  Filter Alerts/1(Trigger) -> Trigger/1
  Alert Level/1 -> Filter Alerts/1(Alert Level In)

== system IntegrationTestSim/Pilot/UAS Pilot Model v6 Enabled System ==
  Own State : Inport
  Alert Level : Inport  Port=2
  Trigger : Inport  Port=3
  Guidance : Inport  Port=4
  Max Turn Rt : Inport  Port=5
  Max Vert Rt : Inport  Port=6
  Enable : EnablePort
  Null AircraftEstimate Bus : NullAircraftEstimateBus/Null AircraftEstimate Bus
  UAS Pilot Model Release 6.1 : uas_pilot_model_r6/UAS Pilot Model Release 6.1  dt=dt  operator_enabled=operator_enabled  deterministicMode=deterministicMode  mean_initial_delay=mean_initial_delay  min_initial_delay=min_initial_delay  coord_delay_k=coord_delay_k  coord_delay_theta=coord_delay_theta  coord_delay_min=coord_delay_min  mean_exec_delay=mean_exec_delay  min_exec_delay=min_exec_delay  min_upd_times=min_upd_times  mean_upd_times=mean_upd_times  rng_seed_initial=rng_seed_initial  rng_seed_coord=rng_seed_coord  rng_seed_execution=rng_seed_execution  rng_seed_update=rng_seed_update  prob_follow_min=prob_follow_min  prob_turn_left=prob_turn_left  prob_turn_table=prob_turn  max_hdg_diff=max_hdg_diff  prob_descend=prob_descend  turn_k=turn_k  turn_theta=turn_theta  turn_offset=turn_offset  turn_k_alt=uasPilot_turnK_alt  turn_theta_alt=uasPilot_turnTheta_alt  turn_offset_alt=uasPilot_turnOffset_alt  alt_k=alt_k  alt_theta=alt_theta  alt_offset=alt_offset  rng_seed_horz=rng_seed_horz  rng_seed_vert=rng_seed_vert  rng_seed_horz_vs_vert=rng_seed_horz_vs_vert  mental_filter_samples=0  mental_filter_climb_thresh=0  mental_filter_turn_thresh=0
  Maneuver Flag : Outport
  Hrz Maneuver : Outport  Port=2
  Vrt Maneuver : Outport  Port=3
  wires:
  Own State/1 -> UAS Pilot Model Release 6.1/1
  Max Turn Rt/1 -> UAS Pilot Model Release 6.1/6
  Max Vert Rt/1 -> UAS Pilot Model Release 6.1/7
  UAS Pilot Model Release 6.1/3 -> Vrt Maneuver/1
  UAS Pilot Model Release 6.1/2 -> Hrz Maneuver/1
  Alert Level/1 -> UAS Pilot Model Release 6.1/3
  Guidance/1 -> UAS Pilot Model Release 6.1/5
  Trigger/1 -> UAS Pilot Model Release 6.1/4
  UAS Pilot Model Release 6.1/1 -> Maneuver Flag/1
  Null AircraftEstimate Bus/1 -> UAS Pilot Model Release 6.1/2

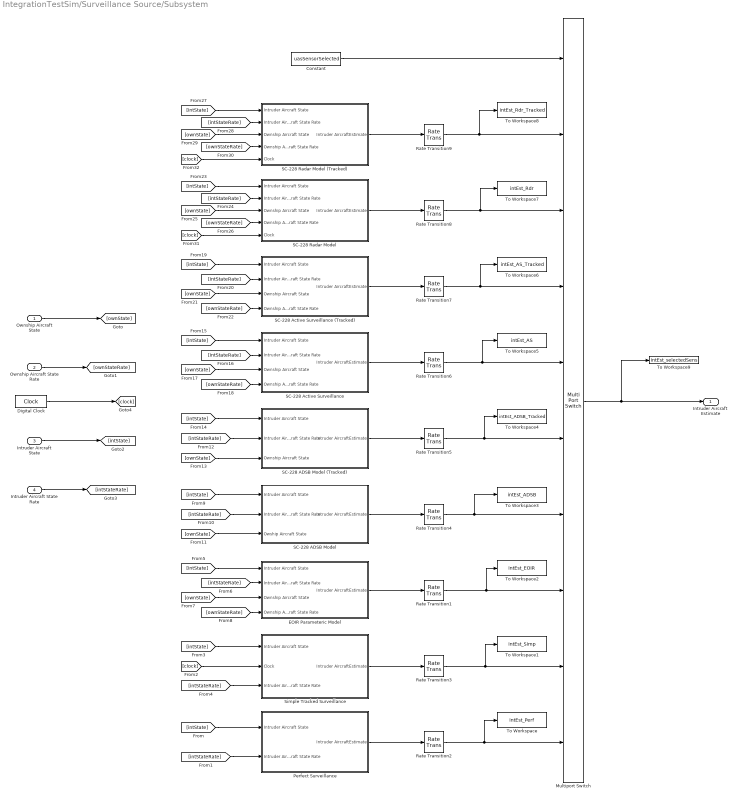
== system IntegrationTestSim/Surveillance Source/Subsystem ==
  Ownship Aircraft State : Inport
  Ownship Aircraft State Rate : Inport  Port=2
  Intruder Aircraft State : Inport  Port=3
  Intruder Aircraft State Rate : Inport  Port=4
  Constant : Constant  Value=uasSensorSelected
  Digital Clock : DigitalClock  SampleTime=uasSurveillance_sampleTime
  EOIR Parameteric Model : Subsystem
  Multiport Switch : MultiPortSwitch  DataPortOrder=Specify indices  DataPortIndices={9,8,7,6,5,4,3,2,1}
  Perfect Surveillance : Subsystem
  Rate Transition{1..9} (9 alike) : RateTransition  OutPortSampleTime=uasSurveillance_sampleTime
  SC-228 ADSB Model : Subsystem
  SC-228 ADSB Model (Tracked) : Subsystem
  SC-228 Active Surveillance : Subsystem
  SC-228 Active Surveillance (Tracked) : Subsystem
  SC-228 Radar Model : Subsystem
  SC-228 Radar Model (Tracked) : Subsystem
  Simple Tracked Surveillance : Subsystem
  To Workspace : ToWorkspace  VariableName=intEst_Perf  SaveFormat=Timeseries  SampleTime=-1
  To Workspace1 : ToWorkspace  VariableName=intEst_Simp  SaveFormat=Timeseries  SampleTime=-1
  To Workspace2 : ToWorkspace  VariableName=intEst_EOIR  SaveFormat=Timeseries  SampleTime=-1
  To Workspace3 : ToWorkspace  VariableName=intEst_ADSB  SaveFormat=Timeseries  SampleTime=-1
  To Workspace4 : ToWorkspace  VariableName=intEst_ADSB_Tracked  SaveFormat=Timeseries  SampleTime=-1
  To Workspace5 : ToWorkspace  VariableName=intEst_AS  SaveFormat=Timeseries  SampleTime=-1
  To Workspace6 : ToWorkspace  VariableName=intEst_AS_Tracked  SaveFormat=Timeseries  SampleTime=-1
  To Workspace7 : ToWorkspace  VariableName=intEst_Rdr  SaveFormat=Timeseries  SampleTime=-1
  To Workspace8 : ToWorkspace  VariableName=intEst_Rdr_Tracked  SaveFormat=Timeseries  SampleTime=-1
  To Workspace9 : ToWorkspace  VariableName=intEst_selectedSens  SaveFormat=Timeseries  SampleTime=-1
  Intruder Aircraft Estimate : Outport
  wires:
  Constant/1 -> Multiport Switch/1
  Multiport Switch/1 -> To Workspace9/1, Intruder Aircraft Estimate/1
  Ownship Aircraft State/1 -> [ownState]
  Ownship Aircraft State Rate/1 -> [ownStateRate]
  Intruder Aircraft State/1 -> [intState]
  Intruder Aircraft State Rate/1 -> [intStateRate]
  [intState] -> Perfect Surveillance/1(Intruder Aircraft State)
  [intStateRate] -> Perfect Surveillance/2(Intruder Aircraft State Rate)
  Perfect Surveillance/1(Intruder AircraftEstimate) -> Rate Transition2/1
  Digital Clock/1 -> [clock]
  [clock] -> Simple Tracked Surveillance/2(Clock)
  [intState] -> Simple Tracked Surveillance/1(Intruder Aircraft State)
  [intStateRate] -> Simple Tracked Surveillance/3(Intruder Aircraft State Rate)
  [intState] -> EOIR Parameteric Model/1(Intruder Aircraft State)
  [intStateRate] -> EOIR Parameteric Model/2(Intruder Aircraft State Rate)
  [ownState] -> EOIR Parameteric Model/3(Ownship Aircraft State)
  [ownStateRate] -> EOIR Parameteric Model/4(Ownship Aircraft State Rate)
  [intState] -> SC-228 ADSB Model/1(Intruder Aircraft State)
  [intStateRate] -> SC-228 ADSB Model/2(Intruder Aircraft State Rate)
  [ownState] -> SC-228 ADSB Model/3(Owship Aircraft State)
  [intState] -> SC-228 ADSB Model (Tracked)/1(Intruder Aircraft State)
  [intStateRate] -> SC-228 ADSB Model (Tracked)/2(Intruder Aircraft State Rate)
  [ownState] -> SC-228 ADSB Model (Tracked)/3(Ownship Aircraft State)
  [intState] -> SC-228 Active Surveillance/1(Intruder Aircraft State)
  [intStateRate] -> SC-228 Active Surveillance/2(Intruder Aircraft State Rate)
  [ownState] -> SC-228 Active Surveillance/3(Ownship Aircraft State)
  [ownStateRate] -> SC-228 Active Surveillance/4(Ownship Aircraft State Rate)
  [intState] -> SC-228 Active Surveillance (Tracked)/1(Intruder Aircraft State)
  [ownState] -> SC-228 Active Surveillance (Tracked)/3(Ownship Aircraft State)
  [intStateRate] -> SC-228 Active Surveillance (Tracked)/2(Intruder Aircraft State Rate)
  [ownStateRate] -> SC-228 Active Surveillance (Tracked)/4(Ownship Aircraft State Rate)
  [intState] -> SC-228 Radar Model/1(Intruder Aircraft State)
  [ownState] -> SC-228 Radar Model/3(Ownship Aircraft State)
  [intStateRate] -> SC-228 Radar Model/2(Intruder Aircraft State Rate)
  [ownStateRate] -> SC-228 Radar Model/4(Ownship Aircraft State Rate)
  [ownState] -> SC-228 Radar Model (Tracked)/3(Ownship Aircraft State)
  [intState] -> SC-228 Radar Model (Tracked)/1(Intruder Aircraft State)
  [intStateRate] -> SC-228 Radar Model (Tracked)/2(Intruder Aircraft State Rate)
  [ownStateRate] -> SC-228 Radar Model (Tracked)/4(Ownship Aircraft State Rate)
  [clock] -> SC-228 Radar Model/5(Clock)
  [clock] -> SC-228 Radar Model (Tracked)/5(Clock)
  Simple Tracked Surveillance/1(Intruder AircraftEstimate) -> Rate Transition3/1
  EOIR Parameteric Model/1(Intruder AircraftEstimate) -> Rate Transition1/1
  SC-228 ADSB Model/1(Intruder AircraftEstimate) -> Rate Transition4/1
  Rate Transition4/1 -> To Workspace3/1, Multiport Switch/7
  Rate Transition1/1 -> To Workspace2/1, Multiport Switch/8
  Rate Transition3/1 -> To Workspace1/1, Multiport Switch/9
  Rate Transition2/1 -> To Workspace/1, Multiport Switch/10
  SC-228 ADSB Model (Tracked)/1(Intruder AircraftEstimate) -> Rate Transition5/1
  Rate Transition5/1 -> To Workspace4/1, Multiport Switch/6
  SC-228 Active Surveillance/1(Intruder AircraftEstimate) -> Rate Transition6/1
  Rate Transition6/1 -> To Workspace5/1, Multiport Switch/5
  SC-228 Active Surveillance (Tracked)/1(Intruder AircraftEstimate) -> Rate Transition7/1
  Rate Transition7/1 -> To Workspace6/1, Multiport Switch/4
  SC-228 Radar Model/1(Intruder AircraftEstimate) -> Rate Transition8/1
  Rate Transition8/1 -> To Workspace7/1, Multiport Switch/3
  SC-228 Radar Model (Tracked)/1(Intruder AircraftEstimate) -> Rate Transition9/1
  Rate Transition9/1 -> To Workspace8/1, Multiport Switch/2
